simulink model "linear_tire_model"  (R2022b)
settings: Solver=VariableStepAuto  StartTime=0.0  StopTime=sim_time  RelTol=1e-3
values from neighbouring files (symbols this model uses):
  Csa = 500    [lineartiremodel.m]
  Cx = 50000    [lineartiremodel.m]
  Cy = 30000    [lineartiremodel.m]
libraries: simulink x2
settings Model: Creator=FATMANURATA  LastModifiedBy=FATMANURATA

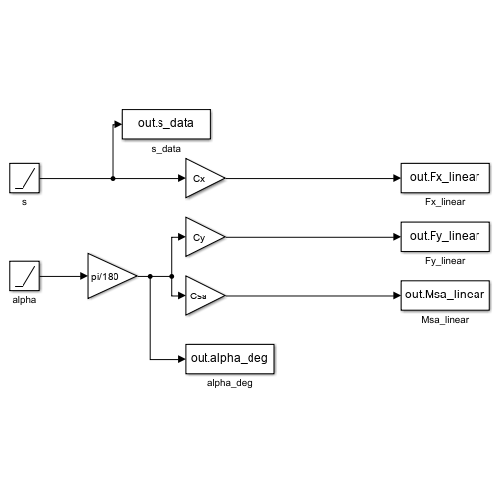
[thumbnail: Simulink's stored preview of the top-level diagram]
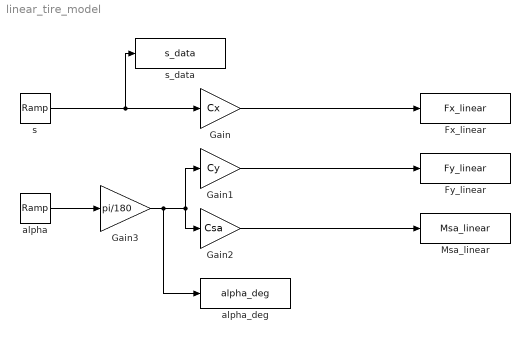
== system linear_tire_model ==
  Fx_linear : ToWorkspace  VariableName=Fx_linear  SampleTime=-1
  Fy_linear : ToWorkspace  VariableName=Fy_linear  SampleTime=-1
  Gain : Gain  Gain=Cx
  Gain1 : Gain  Gain=Cy
  Gain2 : Gain  Gain=Csa
  Gain3 : Gain  Gain=pi/180
  Msa_linear : ToWorkspace  VariableName=Msa_linear  SampleTime=-1
  alpha : simulink/Sources/Ramp  slope=1  start=0  InitialOutput=0
  alpha_deg : ToWorkspace  VariableName=alpha_deg  SampleTime=-1
  s : simulink/Sources/Ramp  slope=0.02  start=0  InitialOutput=0
  s_data : ToWorkspace  VariableName=s_data  SampleTime=-1
  wires:
  s/1 -> s_data/1, Gain/1
  alpha/1 -> Gain3/1
  Gain/1 -> Fx_linear/1
  Gain1/1 -> Fy_linear/1
  Gain2/1 -> Msa_linear/1
  Gain3/1 -> alpha_deg/1, Gain1/1, Gain2/1
